simulink model "LinkageC"  (R2025b)
settings: Solver=VariableStepAuto  StartTime=0  StopTime=numPeriods*T  RelTol=1e-3  AbsTol=1e-3
values from neighbouring files (symbols this model uses):
  A_G = 56.801    [LinkageGeometrySetUp.m]    (also in LinkageGeometrySetUp_imp.m = 55; LinkageGeometry_Fabio_ver.m = 20)
  alpha_0 = deg2rad(0.5)    [Iteration.m]    (also in Iteration_geometry.m; StartUp.m)
  alpha_stall_static = deg2rad(13)    [Iteration.m]    (also in Iteration_geometry.m; StartUp.m)
  AR = b^2/A    [LinkageGeometry_Modify.m]    (also in StartUp.m)
  Cd_cf = 1.5    [Iteration.m]    (also in Iteration_geometry.m; StartUp.m)
  CordOut = linspace(CordOut_root, CordOut_tip, WingSecNum_Out)    [LinkageGeometry_Modify.m]    (also in StartUp.m)
  D = 0;" newline      "    return;" newline      "end" newline      "q = 0.5*rho*Vmag^2;" newline      "D = q*S*CD;" newline      "L = q*S*CL;" newline      "    [build_wing_template.m]
  del_t = t_tot/(numSample)    [InputSetUp.m]
  eta_s = 0.90    (= 0.9)    [Iteration.m]    (also in Iteration_geometry.m; StartUp.m)
  InboardCord = 0.35*L_D/0.037    [LinkageGeometry_Modify.m]    (also in StartUp.m = 0.4)
  k_inboard = k * InboardCord/meanCord    [LinkageGeometry_Modify.m]    (also in StartUp.m = 12.5663706144)
  k_outboard = k * CordOut/meanCord    [LinkageGeometry_Modify.m]    (also in StartUp.m)
  Ka = 10    [StartUp3_control.m]
  Km = 73    [StartUp3_control.m]
  L_C = (3.589/1.5)*L_D    [LinkageGeometrySetUp.m]    (also in LinkageGeometrySetUp_imp.m = (9.37/3.7)*L_D; LinkageGeometry_Fabio_ver.m = 0.07885)
  L_C1 = (2.445/1.5)*L_D    [LinkageGeometrySetUp.m]    (also in LinkageGeometrySetUp_imp.m = (5.91/3.7)*L_D; LinkageGeometry_Fabio_ver.m = 0.04893)
  L_D = L_D_val(iter)    [Iteration_geometry.m]    (also in LinkageGeometry_Fabio_ver.m = 0.03019; StartUp.m = 0.037)
  L_EF = (1.494/1.5)*L_D    [LinkageGeometrySetUp.m]    (also in LinkageGeometrySetUp_imp.m = (4.468/3.7)*L_D; LinkageGeometry_Fabio_ver.m = 0.036)
  L_EG = (1.265/1.5)*L_D    [LinkageGeometrySetUp.m]    (also in LinkageGeometrySetUp_imp.m = L_C2; LinkageGeometry_Fabio_ver.m = 0.03)
  L_F = (16.189/1.5)*L_D    [LinkageGeometrySetUp.m]    (also in LinkageGeometrySetUp_imp.m = (39.93/3.7)*L_D; LinkageGeometry_Fabio_ver.m = 0.364)
  L_FH = (1.002/1.5)*L_D    [LinkageGeometrySetUp.m]    (also in LinkageGeometrySetUp_imp.m = (2.842/3.7)*L_D; LinkageGeometry_Fabio_ver.m = 0.02)
  L_Fl = (16.118/1.5)*L_D    [LinkageGeometrySetUp.m]    (also in LinkageGeometrySetUp_imp.m = L_F; LinkageGeometry_Fabio_ver.m = 0.364)
  L_Fp = (4.051/1.5)*L_D    [LinkageGeometrySetUp.m]    (also in LinkageGeometrySetUp_imp.m = (9.99/3.7)*L_D; LinkageGeometry_Fabio_ver.m = 0.14288)
  L_GH = (1.129/1.5)*L_D    [LinkageGeometrySetUp.m]    (also in LinkageGeometrySetUp_imp.m = (3.046/3.7)*L_D; LinkageGeometry_Fabio_ver.m = 0.016)
  L_t = 0.5/100    (= 0.005)    [LinkageGeometrySetUp.m]    (also in LinkageGeometrySetUp_imp.m; LinkageGeometry_Fabio_ver.m; LinkageGeometry_Modify.m)
  L_tip = (19.334/1.5)*L_D    [LinkageGeometrySetUp.m]    (also in LinkageGeometrySetUp_imp.m = (43/3.7)*L_D; LinkageGeometry_Fabio_ver.m = 0.55)
  M_in_i = M_in/WingSecNum_In    (= 0.0341666666667)    [StartUp.m]
  M_ser = 0.02    [StartUp.m]
  mu = 1.81e-5    (= 1.81e-05)    [Iteration.m]    (also in Iteration_geometry.m; StartUp.m)
  noise_freq_cutoff = 20*ang_freq    [InputSetUp.m]
  P_ref = 10    [StartUp3_control.m]
  phase_data_lookup = phase_data_lookup(1:(end-1))    [StartUp.m]
  pitch_data_lookup = pitch_ts.Data(1:numSampPerT)    [InputSetUp.m]
  pitch_gain = linspace(0.1, 1, WingSecNum_Out)    [InputSetUp.m]
  pitch_lookup_input = 1    [Iteration.m]    (also in Iteration_geometry.m; StartUp.m)
  pitch_mean = deg2rad(20)    [Iteration.m]    (also in Iteration_geometry.m; Iteration_speed.m; StartUp.m = deg2rad(1); StartUp3_control.m = deg2rad(1))
  rho = 1.225    [StartUp.m]
  SectionWidth_In = L_Inboard/WingSecNum_In    [LinkageGeometry_Modify.m]    (also in StartUp.m = (L_Inboard/WingSecNum_In)*0.6)
  SectionWidth_Out = L_outboard/WingSecNum_Out    [LinkageGeometry_Modify.m]    (also in StartUp.m)
  SpeedControlYes = 1    [StartUp3_control.m]
  TorqueLimit = 7.2    [StartUp3_control.m]
  U = 0.1    [Iteration.m]    (also in Iteration_geometry.m; StartUp.m)
  xi = 0.0    (= 0)    [Iteration.m]    (also in Iteration_geometry.m; StartUp.m)
undefined symbols (not defined in the file or in its folder): angle_data_lookup, DiscIntNeverNeededParam, magnitude, Pivot, X, Y, Z
libraries: sm_lib x1370, nesl_utility x916, simulink x478, cstblocks x78, simulink_extras x10, slpidlib x2
(part 14 of 57)

== system LinkageC/Subsystem/Wing Tip/Angle ==
  PS-Simulink Converter{1..4} (4 alike) : nesl_utility/PS-Simulink Converter  PhysicalDomain=network_engine_domain  SubClassName=ps_output  LeftPortType=input  RightPortType=output  PseudoPeriodic=off  Frequencies=[]  VectorFormat=inherit  Unit=inherit  AffineConversion=off
  Radians to Degrees : simulink_extras/Transformations/Radians to Degrees
  Subtract : Sum  Inputs=+-
  Subtract1 : Sum  Inputs=+-
  To Workspace : ToWorkspace  VariableName=simout6  SampleTime=-1
  Transform Sensor : sm_lib/Frames and Transforms/Transform Sensor  MeasurementFrame=World  RotationSequence=XYX  SenseAngle=off  SenseAxis=off  SenseQ=off  SenseR=off  SenseRotationSequence=off  SenseOmegaX=off  SenseOmegaY=off  SenseOmegaZ=off  SenseOmega=off  SenseQDot=off  SenseRDot=off  SenseRotationSequenceDot=off  SenseAlphaX=off  SenseAlphaY=off  SenseAlphaZ=off  SenseAlpha=off  SenseQDDot=off  SenseRDDot=off  SenseX=on  SenseY=on  SenseZ=off  SenseXYZ=off  SenseRad=off  SenseAzim=off  SenseDist=off  SenseInc=off  SenseXDot=off  SenseYDot=off  SenseZDot=off  SenseXYZDot=off  SenseRadDot=off  SenseAzimDot=off  SenseDistDot=off  SenseIncDot=off  SenseXDDot=off  SenseYDDot=off  SenseZDDot=off  SenseXYZDDot=off  SenseRadDDot=off  SenseAzimDDot=off  SenseDistDDot=off  SenseIncDDot=off
  Transform Sensor1 : sm_lib/Frames and Transforms/Transform Sensor  MeasurementFrame=World  RotationSequence=XYX  SenseAngle=off  SenseAxis=off  SenseQ=off  SenseR=off  SenseRotationSequence=off  SenseOmegaX=off  SenseOmegaY=off  SenseOmegaZ=off  SenseOmega=off  SenseQDot=off  SenseRDot=off  SenseRotationSequenceDot=off  SenseAlphaX=off  SenseAlphaY=off  SenseAlphaZ=off  SenseAlpha=off  SenseQDDot=off  SenseRDDot=off  SenseX=on  SenseY=on  SenseZ=off  SenseXYZ=off  SenseRad=off  SenseAzim=off  SenseDist=off  SenseInc=off  SenseXDot=off  SenseYDot=off  SenseZDot=off  SenseXYZDot=off  SenseRadDot=off  SenseAzimDot=off  SenseDistDot=off  SenseIncDot=off  SenseXDDot=off  SenseYDDot=off  SenseZDDot=off  SenseXYZDDot=off  SenseRadDDot=off  SenseAzimDDot=off  SenseDistDDot=off  SenseIncDDot=off
  Trigonometric Function : Trigonometry  Operator=atan2
  World Frame : sm_lib/Frames and Transforms/World Frame
  Pivot : PMIOPort  Side=Right
  Other Frame : PMIOPort  Port=2  Side=Right
  wires:
  Subtract/1 -> Trigonometric Function/2
  PS-Simulink Converter2/1 -> Subtract1/1
  Radians to Degrees/1 -> To Workspace/1  "OB_deg"
  Subtract1/1 -> Trigonometric Function/1
  PS-Simulink Converter4/1 -> Subtract1/2
  PS-Simulink Converter3/1 -> Subtract/2
  PS-Simulink Converter1/1 -> Subtract/1
  Trigonometric Function/1 -> Radians to Degrees/1
  connections:
  PS-Simulink Converter3/LConn1 -- Transform Sensor1/RConn2
  World Frame/RConn1 -- Transform Sensor/LConn1 -- Transform Sensor1/LConn1
  Transform Sensor/RConn3 -- PS-Simulink Converter2/LConn1
  PS-Simulink Converter1/LConn1 -- Transform Sensor/RConn2
  Transform Sensor1/RConn3 -- PS-Simulink Converter4/LConn1
  Transform Sensor/RConn1 -- Other Frame/RConn1
  Transform Sensor1/RConn1 -- Pivot/RConn1

== system LinkageC/Subsystem/Wing Tip/LinkEF_discrete ==
  Subsystem : Subsystem
  Subsystem1 : Subsystem
  Subsystem2 : Subsystem
  Subsystem3 : Subsystem
  Subsystem4 : Subsystem
  Conn1 : PMIOPort  Side=Left
  Conn2 : PMIOPort  Port=2  Side=Right
  connections:
  Subsystem4/RConn1 -- Conn2/RConn1
  Subsystem/LConn1 -- Conn1/RConn1
  Subsystem2/LConn1 -- Subsystem1/RConn1
  Subsystem/RConn1 -- Subsystem1/LConn1
  Subsystem2/RConn1 -- Subsystem3/LConn1
  Subsystem4/LConn1 -- Subsystem3/RConn1

== system LinkageC/Subsystem/Wing Tip/LinkGH_discrete ==
  LinkGH_0 : Subsystem
  LinkGH_1 : Subsystem
  LinkGH_2 : Subsystem
  LinkGH_3 : Subsystem
  LinkGH_4 : Subsystem
  Pin G Pos : PMIOPort  Side=Left
  Conn2 : PMIOPort  Port=2  Side=Right
  connections:
  LinkGH_3/LConn1 -- LinkGH_2/RConn1
  LinkGH_1/RConn1 -- LinkGH_2/LConn1
  LinkGH_0/LConn1 -- Pin G Pos/RConn1
  LinkGH_3/RConn1 -- LinkGH_4/LConn1
  LinkGH_4/RConn1 -- Conn2/RConn1
  LinkGH_0/RConn1 -- LinkGH_1/LConn1

== system LinkageC/Subsystem/Wing Tip/WingSeg_Out_1 ==
  1993dL&dT : Subsystem
      settings: PortSchema="{\"entries\":[{\"content\":{\"sides\":[{\"content\":{\"connectorIds\":[\"In1\",\"In2\"]},\"type\":\"ConnectorPlacement.EquallySpacedRectSide\",\"uuid\":\"e65777f2-64e1-48f2-8a97-1c4430d49e8c\"},{\"content\":{\"connectorIds\":[\"Out1\",\"Out2\"],\"side\":\"RIGHT\"},\"type\":\"ConnectorPlacement.EquallySpacedRectSide\",\"uuid\":\"b36152b1-49d2-4fe8-8958-784e9c481724\"},{\"content\":{\"connectorIds\":[\"LConn1\"],\"side\":\"TOP\"},\"type\":\"ConnectorPlacement.EquallySpacedRectSide\",\"uuid\":\"e55ca923-aa34-4679-961a-c06571c550d8\"}]},\"type\":\"ConnectorPlacement.EquallySpacedConnector\",\"uuid\":\"74bedadb-397c-4a7f-b538-7cebaf15bb03\"}],\"packageUris\":[\"http://schema.mathworks.com/mf0/Connector/R2020b\"],\"version\":\"1.0\"}"
  Discrete Derivative : simulink/Discrete/Discrete Derivative  gainval=1.0  ICPrevScaledInput=0.0  OutMin=[]  OutMax=[]  OutDataType=fixdt(1, 16)  OutScaling=2^-10  DoSatur=off
  Discrete Derivative1 : simulink/Discrete/Discrete Derivative  gainval=1.0  ICPrevScaledInput=0.0  OutMin=[]  OutMax=[]  OutDataType=fixdt(1, 16)  OutScaling=2^-10  DoSatur=off
  DocBlock : simulink/Model-Wide Utilities/DocBlock  DocumentType=Text
      content=|
      | For each wing section, things that need to be specified includes:
      | - Wing solid dimension (use wing modify script)
      | - Wing joint gain (pitchGain, pitchGain1, pitchGain2)
      | - PivotXfm & COMXfm
      | - i value
      | - inboard_yes?
  In_yes : Constant  Value=0
  Product : Product
  Switch : Switch  Criteria=u2 > Threshold  SaturateOnIntegerOverflow=off  InputSameDT=off
  WingSolid : sm_lib/Body Elements/Brick Solid  BrickDimensions=[0.35, L_t, SectionWidth_Out]  BrickDimensionsUnits=m  ExportEntireGeometry=off  InertiaType=CalculateFromGeometry  BasedOnType=Mass  Density=1000  DensityUnits=kg/m^3  Mass=0.031429  MassUnits=kg  CenterOfMass=[0 0 0]  CenterOfMassUnits=m  MomentsOfInertia=[1 1 1]  MomentsOfInertiaUnits=kg*m^2  ProductsOfInertia=[0 0 0]  ProductsOfInertiaUnits=kg*m^2  GraphicType=FromGeometry  MarkerShape=Sphere  MarkerSize=10  GraphicVisPropType=SimpleVisualProperties  GraphicDiffuseColor=[0.37 0.4 0.8]  GraphicOpacity=1  GraphicSpecularColor=[0.5 0.5 0.5 1.0]  GraphicAmbientColor=[0.15 0.15 0.15 1.0]  GraphicEmissiveColor=[0.0 0.0 0.0 1.0]  GraphicShininess=75  DoExposeReferenceFrame=on  SerializedFrames=<Frames/>
  Wing_Joint : sm_lib/Joints/Revolute Joint  JointMode=Normal  CompositeWrenchDir=FollowerOnBase  CompositeWrenchFrame=BaseFrame  SenseConstraintForce=off  SenseConstraintTorque=off  SenseTotalForce=off  SenseTotalTorque=off  PositionTargetSpecify=off  PositionTargetPriority=High  PositionTargetValue=0  PositionTargetValueUnits=deg  VelocityTargetSpecify=off  VelocityTargetPriority=High  VelocityTargetValue=0  VelocityTargetValueUnits=deg/s  EquilibriumPosition=0  EquilibriumPositionUnits=deg  SpringStiffness=0  SpringStiffnessUnits=N*m/deg  DampingCoefficient=dampingOfJoints  DampingCoefficientUnits=N*m/(deg/s)  LowerLimitSpecify=off  LowerLimitBound=-90  LowerLimitBoundUnits=deg  LowerLimitStiffness=1e4  LowerLimitStiffnessUnits=N*m/deg  LowerLimitDamping=10  LowerLimitDampingUnits=N*m/(deg/s)  LowerLimitTransitionRegionWidth=0.1  LowerLimitTransitionRegionWidthUnits=deg  UpperLimitSpecify=off  UpperLimitBound=90  UpperLimitBoundUnits=deg  UpperLimitStiffness=1e4  UpperLimitStiffnessUnits=N*m/deg  UpperLimitDamping=10  UpperLimitDampingUnits=N*m/(deg/s)  UpperLimitTransitionRegionWidth=0.1  UpperLimitTransitionRegionWidthUnits=deg  TorqueActuationMode=ComputedTorque  MotionActuationMode=InputMotion  SensePosition=off  SenseVelocity=off  SenseAcceleration=off  SenseTorqueForce=off  SenseLowerLimitTorqueForce=off  SenseUpperLimitTorqueForce=off
  Xfm : sm_lib/Frames and Transforms/Rigid Transform  RotationMethod=None  FollAlignAxisA=+X  BaseAlignAxisA=+Y  FollAlignAxisB=+Y  BaseAlignAxisB=+Z  RotationStandardAxis=+Z  RotationAngle=0  RotationAngleUnits=deg  RotationArbitraryAxis=[0 0 1]  RotationSequenceAxes=FollowerAxes  RotationSequence=XYX  RotationSequenceAngles=[0 0 0]  RotationSequenceAnglesUnits=deg  RotationMatrix=[1 0 0;0 1 0;0 0 1]  Quaternion=[1 0 0 0]  TranslationMethod=Cartesian  TranslationCartesianOffset=[0.0875 0 0.03]  TranslationCartesianOffsetUnits=m  TranslationStandardAxis=+Z  TranslationStandardOffset=0  TranslationStandardOffsetUnits=m  TranslationROffset=0  TranslationROffsetUnits=m  TranslationThetaOffset=0  TranslationThetaOffsetUnits=deg  TranslationZOffset=0  TranslationZOffsetUnits=m
  i : Constant
  pitchGain : Gain  Gain=0.1
  pitchGain1 : Gain  Gain=0.1
  pitchGain2 : Gain  Gain=0.1
  pitchPS : nesl_utility/Simulink-PS Converter  PhysicalDomain=network_engine_domain  SubClassName=ps_input  LeftPortType=input  RightPortType=output  PseudoPeriodic=off  Frequencies=[]  NoiseDistribution=none  NoiseParameters=[]  Unit=rad  AffineConversion=off  FilteringAndDerivatives=provide  SimscapeFilterOrder=1  InputFilterTimeConstant=0.001  UdotUserProvided=2
  pitch_lookup?(1=yes) : Constant  Value=pitch_lookup_input
  pitch_tip_in : FromWorkspace  VariableName=pitch_tip_in  SampleTime=del_t
  simulation sign convention differ : Constant  Value=-1
  WingRef_Frame : PMIOPort  Side=Left
  dL : Outport
  dT : Outport  Port=2
  wires:
  pitch_tip_in/1 -> Switch/3  "pitch"
  [pitch_m] -> Switch/1
  Switch/1 -> Product/1
  pitch_lookup?(1=yes)/1 -> Switch/2
  Product/1 -> pitchGain/1, Discrete Derivative/1
  simulation sign convention differ/1 -> Product/2
  In_yes/1 -> 1993dL&dT/2(inboard_yes?)
  i/1 -> 1993dL&dT/1(i)
  1993dL&dT/2(dT) -> dT/1
  Discrete Derivative/1 -> pitchGain1/1, Discrete Derivative1/1
  pitchGain/1 -> pitchPS/1
  1993dL&dT/1(dL) -> dL/1
  pitchGain2/1 -> pitchPS/3
  Discrete Derivative1/1 -> pitchGain2/1  "acc"
  pitchGain1/1 -> pitchPS/2
  connections:
  Xfm/LConn1 -- Wing_Joint/RConn1
  1993dL&dT/LConn1 -- Xfm/RConn1 -- WingSolid/RConn1
  pitchPS/RConn1 -- Wing_Joint/LConn2
  Wing_Joint/LConn1 -- WingRef_Frame/RConn1

== system LinkageC/Subsystem/Wing Tip/WingSeg_Out_10 ==
  1993dL&dT : Subsystem
      settings: PortSchema="{\"entries\":[{\"content\":{\"sides\":[{\"content\":{\"connectorIds\":[\"In1\",\"In2\"]},\"type\":\"ConnectorPlacement.EquallySpacedRectSide\",\"uuid\":\"e65777f2-64e1-48f2-8a97-1c4430d49e8c\"},{\"content\":{\"connectorIds\":[\"Out1\",\"Out2\"],\"side\":\"RIGHT\"},\"type\":\"ConnectorPlacement.EquallySpacedRectSide\",\"uuid\":\"b36152b1-49d2-4fe8-8958-784e9c481724\"},{\"content\":{\"connectorIds\":[\"LConn1\"],\"side\":\"TOP\"},\"type\":\"ConnectorPlacement.EquallySpacedRectSide\",\"uuid\":\"e55ca923-aa34-4679-961a-c06571c550d8\"}]},\"type\":\"ConnectorPlacement.EquallySpacedConnector\",\"uuid\":\"74bedadb-397c-4a7f-b538-7cebaf15bb03\"}],\"packageUris\":[\"http://schema.mathworks.com/mf0/Connector/R2020b\"],\"version\":\"1.0\"}"
  Discrete Derivative : simulink/Discrete/Discrete Derivative  gainval=1.0  ICPrevScaledInput=0.0  OutMin=[]  OutMax=[]  OutDataType=fixdt(1, 16)  OutScaling=2^-10  DoSatur=off
  Discrete Derivative1 : simulink/Discrete/Discrete Derivative  gainval=1.0  ICPrevScaledInput=0.0  OutMin=[]  OutMax=[]  OutDataType=fixdt(1, 16)  OutScaling=2^-10  DoSatur=off
  DocBlock : simulink/Model-Wide Utilities/DocBlock  DocumentType=Text
      content=|
      | For each wing section, things that need to be specified includes:
      | - Wing solid dimension (use wing modify script)
      | - Wing joint gain (pitchGain, pitchGain1, pitchGain2)
      | - PivotXfm & COMXfm
      | - i value
      | - inboard_yes?
  In_yes : Constant  Value=0
  Product : Product
  Switch : Switch  Criteria=u2 > Threshold  SaturateOnIntegerOverflow=off  InputSameDT=off
  WingSolid : sm_lib/Body Elements/Brick Solid  BrickDimensions=[0.14, L_t, SectionWidth_Out]  BrickDimensionsUnits=m  ExportEntireGeometry=off  InertiaType=CalculateFromGeometry  BasedOnType=Mass  Density=1000  DensityUnits=kg/m^3  Mass=0.012571  MassUnits=kg  CenterOfMass=[0 0 0]  CenterOfMassUnits=m  MomentsOfInertia=[1 1 1]  MomentsOfInertiaUnits=kg*m^2  ProductsOfInertia=[0 0 0]  ProductsOfInertiaUnits=kg*m^2  GraphicType=FromGeometry  MarkerShape=Sphere  MarkerSize=10  GraphicVisPropType=SimpleVisualProperties  GraphicDiffuseColor=[1 0.4 0.8]  GraphicOpacity=1  GraphicSpecularColor=[0.5 0.5 0.5 1.0]  GraphicAmbientColor=[0.15 0.15 0.15 1.0]  GraphicEmissiveColor=[0.0 0.0 0.0 1.0]  GraphicShininess=75  DoExposeReferenceFrame=on  SerializedFrames=<Frames/>
  Wing_Joint : sm_lib/Joints/Revolute Joint  JointMode=Normal  CompositeWrenchDir=FollowerOnBase  CompositeWrenchFrame=BaseFrame  SenseConstraintForce=off  SenseConstraintTorque=off  SenseTotalForce=off  SenseTotalTorque=off  PositionTargetSpecify=off  PositionTargetPriority=High  PositionTargetValue=0  PositionTargetValueUnits=deg  VelocityTargetSpecify=off  VelocityTargetPriority=High  VelocityTargetValue=0  VelocityTargetValueUnits=deg/s  EquilibriumPosition=0  EquilibriumPositionUnits=deg  SpringStiffness=0  SpringStiffnessUnits=N*m/deg  DampingCoefficient=dampingOfJoints  DampingCoefficientUnits=N*m/(deg/s)  LowerLimitSpecify=off  LowerLimitBound=-90  LowerLimitBoundUnits=deg  LowerLimitStiffness=1e4  LowerLimitStiffnessUnits=N*m/deg  LowerLimitDamping=10  LowerLimitDampingUnits=N*m/(deg/s)  LowerLimitTransitionRegionWidth=0.1  LowerLimitTransitionRegionWidthUnits=deg  UpperLimitSpecify=off  UpperLimitBound=90  UpperLimitBoundUnits=deg  UpperLimitStiffness=1e4  UpperLimitStiffnessUnits=N*m/deg  UpperLimitDamping=10  UpperLimitDampingUnits=N*m/(deg/s)  UpperLimitTransitionRegionWidth=0.1  UpperLimitTransitionRegionWidthUnits=deg  TorqueActuationMode=ComputedTorque  MotionActuationMode=InputMotion  SensePosition=off  SenseVelocity=off  SenseAcceleration=off  SenseTorqueForce=off  SenseLowerLimitTorqueForce=off  SenseUpperLimitTorqueForce=off
  Xfm : sm_lib/Frames and Transforms/Rigid Transform  RotationMethod=None  FollAlignAxisA=+X  BaseAlignAxisA=+Y  FollAlignAxisB=+Y  BaseAlignAxisB=+Z  RotationStandardAxis=+Z  RotationAngle=0  RotationAngleUnits=deg  RotationArbitraryAxis=[0 0 1]  RotationSequenceAxes=FollowerAxes  RotationSequence=XYX  RotationSequenceAngles=[0 0 0]  RotationSequenceAnglesUnits=deg  RotationMatrix=[1 0 0;0 1 0;0 0 1]  Quaternion=[1 0 0 0]  TranslationMethod=Cartesian  TranslationCartesianOffset=[0.035 0 0.57]  TranslationCartesianOffsetUnits=m  TranslationStandardAxis=+Z  TranslationStandardOffset=0  TranslationStandardOffsetUnits=m  TranslationROffset=0  TranslationROffsetUnits=m  TranslationThetaOffset=0  TranslationThetaOffsetUnits=deg  TranslationZOffset=0  TranslationZOffsetUnits=m
  i : Constant  Value=10
  pitchGain : Gain
  pitchGain1 : Gain
  pitchGain2 : Gain
  pitchPS : nesl_utility/Simulink-PS Converter  PhysicalDomain=network_engine_domain  SubClassName=ps_input  LeftPortType=input  RightPortType=output  PseudoPeriodic=off  Frequencies=[]  NoiseDistribution=none  NoiseParameters=[]  Unit=rad  AffineConversion=off  FilteringAndDerivatives=provide  SimscapeFilterOrder=1  InputFilterTimeConstant=0.001  UdotUserProvided=2
  pitch_lookup?(1=yes) : Constant  Value=pitch_lookup_input
  pitch_tip_in : FromWorkspace  VariableName=pitch_tip_in  SampleTime=del_t
  simulation sign convention differ : Constant  Value=-1
  WingRef_Frame : PMIOPort  Side=Left
  dL : Outport
  dT : Outport  Port=2
  wires:
  pitch_tip_in/1 -> Switch/3  "pitch"
  [pitch_m] -> Switch/1
  Switch/1 -> Product/1
  pitch_lookup?(1=yes)/1 -> Switch/2
  Product/1 -> pitchGain/1, Discrete Derivative/1
  simulation sign convention differ/1 -> Product/2
  In_yes/1 -> 1993dL&dT/2(inboard_yes?)
  i/1 -> 1993dL&dT/1(i)
  1993dL&dT/2(dT) -> dT/1
  Discrete Derivative/1 -> pitchGain1/1, Discrete Derivative1/1
  pitchGain/1 -> pitchPS/1
  1993dL&dT/1(dL) -> dL/1
  pitchGain2/1 -> pitchPS/3
  Discrete Derivative1/1 -> pitchGain2/1  "acc"
  pitchGain1/1 -> pitchPS/2
  connections:
  Xfm/LConn1 -- Wing_Joint/RConn1
  1993dL&dT/LConn1 -- Xfm/RConn1 -- WingSolid/RConn1
  pitchPS/RConn1 -- Wing_Joint/LConn2
  Wing_Joint/LConn1 -- WingRef_Frame/RConn1

== system LinkageC/Subsystem/Wing Tip/WingSeg_Out_2 ==
  1993dL&dT : Subsystem
      settings: PortSchema="{\"entries\":[{\"content\":{\"sides\":[{\"content\":{\"connectorIds\":[\"In1\",\"In2\"]},\"type\":\"ConnectorPlacement.EquallySpacedRectSide\",\"uuid\":\"e65777f2-64e1-48f2-8a97-1c4430d49e8c\"},{\"content\":{\"connectorIds\":[\"Out1\",\"Out2\"],\"side\":\"RIGHT\"},\"type\":\"ConnectorPlacement.EquallySpacedRectSide\",\"uuid\":\"b36152b1-49d2-4fe8-8958-784e9c481724\"},{\"content\":{\"connectorIds\":[\"LConn1\"],\"side\":\"TOP\"},\"type\":\"ConnectorPlacement.EquallySpacedRectSide\",\"uuid\":\"e55ca923-aa34-4679-961a-c06571c550d8\"}]},\"type\":\"ConnectorPlacement.EquallySpacedConnector\",\"uuid\":\"74bedadb-397c-4a7f-b538-7cebaf15bb03\"}],\"packageUris\":[\"http://schema.mathworks.com/mf0/Connector/R2020b\"],\"version\":\"1.0\"}"
  Discrete Derivative : simulink/Discrete/Discrete Derivative  gainval=1.0  ICPrevScaledInput=0.0  OutMin=[]  OutMax=[]  OutDataType=fixdt(1, 16)  OutScaling=2^-10  DoSatur=off
  Discrete Derivative1 : simulink/Discrete/Discrete Derivative  gainval=1.0  ICPrevScaledInput=0.0  OutMin=[]  OutMax=[]  OutDataType=fixdt(1, 16)  OutScaling=2^-10  DoSatur=off
  DocBlock : simulink/Model-Wide Utilities/DocBlock  DocumentType=Text
      content=|
      | For each wing section, things that need to be specified includes:
      | - Wing solid dimension (use wing modify script)
      | - Wing joint gain (pitchGain, pitchGain1, pitchGain2)
      | - PivotXfm & COMXfm
      | - i value
      | - inboard_yes?
  In_yes : Constant  Value=0
  Product : Product
  Switch : Switch  Criteria=u2 > Threshold  SaturateOnIntegerOverflow=off  InputSameDT=off
  WingSolid : sm_lib/Body Elements/Brick Solid  BrickDimensions=[0.32667, L_t, SectionWidth_Out]  BrickDimensionsUnits=m  ExportEntireGeometry=off  InertiaType=CalculateFromGeometry  BasedOnType=Mass  Density=1000  DensityUnits=kg/m^3  Mass=0.029333  MassUnits=kg  CenterOfMass=[0 0 0]  CenterOfMassUnits=m  MomentsOfInertia=[1 1 1]  MomentsOfInertiaUnits=kg*m^2  ProductsOfInertia=[0 0 0]  ProductsOfInertiaUnits=kg*m^2  GraphicType=FromGeometry  MarkerShape=Sphere  MarkerSize=10  GraphicVisPropType=SimpleVisualProperties  GraphicDiffuseColor=[0.44 0.4 0.8]  GraphicOpacity=1  GraphicSpecularColor=[0.5 0.5 0.5 1.0]  GraphicAmbientColor=[0.15 0.15 0.15 1.0]  GraphicEmissiveColor=[0.0 0.0 0.0 1.0]  GraphicShininess=75  DoExposeReferenceFrame=on  SerializedFrames=<Frames/>
  Wing_Joint : sm_lib/Joints/Revolute Joint  JointMode=Normal  CompositeWrenchDir=FollowerOnBase  CompositeWrenchFrame=BaseFrame  SenseConstraintForce=off  SenseConstraintTorque=off  SenseTotalForce=off  SenseTotalTorque=off  PositionTargetSpecify=off  PositionTargetPriority=High  PositionTargetValue=0  PositionTargetValueUnits=deg  VelocityTargetSpecify=off  VelocityTargetPriority=High  VelocityTargetValue=0  VelocityTargetValueUnits=deg/s  EquilibriumPosition=0  EquilibriumPositionUnits=deg  SpringStiffness=0  SpringStiffnessUnits=N*m/deg  DampingCoefficient=dampingOfJoints  DampingCoefficientUnits=N*m/(deg/s)  LowerLimitSpecify=off  LowerLimitBound=-90  LowerLimitBoundUnits=deg  LowerLimitStiffness=1e4  LowerLimitStiffnessUnits=N*m/deg  LowerLimitDamping=10  LowerLimitDampingUnits=N*m/(deg/s)  LowerLimitTransitionRegionWidth=0.1  LowerLimitTransitionRegionWidthUnits=deg  UpperLimitSpecify=off  UpperLimitBound=90  UpperLimitBoundUnits=deg  UpperLimitStiffness=1e4  UpperLimitStiffnessUnits=N*m/deg  UpperLimitDamping=10  UpperLimitDampingUnits=N*m/(deg/s)  UpperLimitTransitionRegionWidth=0.1  UpperLimitTransitionRegionWidthUnits=deg  TorqueActuationMode=ComputedTorque  MotionActuationMode=InputMotion  SensePosition=off  SenseVelocity=off  SenseAcceleration=off  SenseTorqueForce=off  SenseLowerLimitTorqueForce=off  SenseUpperLimitTorqueForce=off
  Xfm : sm_lib/Frames and Transforms/Rigid Transform  RotationMethod=None  FollAlignAxisA=+X  BaseAlignAxisA=+Y  FollAlignAxisB=+Y  BaseAlignAxisB=+Z  RotationStandardAxis=+Z  RotationAngle=0  RotationAngleUnits=deg  RotationArbitraryAxis=[0 0 1]  RotationSequenceAxes=FollowerAxes  RotationSequence=XYX  RotationSequenceAngles=[0 0 0]  RotationSequenceAnglesUnits=deg  RotationMatrix=[1 0 0;0 1 0;0 0 1]  Quaternion=[1 0 0 0]  TranslationMethod=Cartesian  TranslationCartesianOffset=[0.081667 0 0.09]  TranslationCartesianOffsetUnits=m  TranslationStandardAxis=+Z  TranslationStandardOffset=0  TranslationStandardOffsetUnits=m  TranslationROffset=0  TranslationROffsetUnits=m  TranslationThetaOffset=0  TranslationThetaOffsetUnits=deg  TranslationZOffset=0  TranslationZOffsetUnits=m
  i : Constant  Value=2
  pitchGain : Gain  Gain=0.2
  pitchGain1 : Gain  Gain=0.2
  pitchGain2 : Gain  Gain=0.2
  pitchPS : nesl_utility/Simulink-PS Converter  PhysicalDomain=network_engine_domain  SubClassName=ps_input  LeftPortType=input  RightPortType=output  PseudoPeriodic=off  Frequencies=[]  NoiseDistribution=none  NoiseParameters=[]  Unit=rad  AffineConversion=off  FilteringAndDerivatives=provide  SimscapeFilterOrder=1  InputFilterTimeConstant=0.001  UdotUserProvided=2
  pitch_lookup?(1=yes) : Constant  Value=pitch_lookup_input
  pitch_tip_in : FromWorkspace  VariableName=pitch_tip_in  SampleTime=del_t
  simulation sign convention differ : Constant  Value=-1
  WingRef_Frame : PMIOPort  Side=Left
  dL : Outport
  dT : Outport  Port=2
  wires:
  pitch_tip_in/1 -> Switch/3  "pitch"
  [pitch_m] -> Switch/1
  Switch/1 -> Product/1
  pitch_lookup?(1=yes)/1 -> Switch/2
  Product/1 -> pitchGain/1, Discrete Derivative/1
  simulation sign convention differ/1 -> Product/2
  In_yes/1 -> 1993dL&dT/2(inboard_yes?)
  i/1 -> 1993dL&dT/1(i)
  1993dL&dT/2(dT) -> dT/1
  Discrete Derivative/1 -> pitchGain1/1, Discrete Derivative1/1
  pitchGain/1 -> pitchPS/1
  1993dL&dT/1(dL) -> dL/1
  pitchGain2/1 -> pitchPS/3
  Discrete Derivative1/1 -> pitchGain2/1  "acc"
  pitchGain1/1 -> pitchPS/2
  connections:
  Xfm/LConn1 -- Wing_Joint/RConn1
  1993dL&dT/LConn1 -- Xfm/RConn1 -- WingSolid/RConn1
  pitchPS/RConn1 -- Wing_Joint/LConn2
  Wing_Joint/LConn1 -- WingRef_Frame/RConn1

== system LinkageC/Subsystem/Wing Tip/WingSeg_Out_3 ==
  1993dL&dT : Subsystem
      settings: PortSchema="{\"entries\":[{\"content\":{\"sides\":[{\"content\":{\"connectorIds\":[\"In1\",\"In2\"]},\"type\":\"ConnectorPlacement.EquallySpacedRectSide\",\"uuid\":\"e65777f2-64e1-48f2-8a97-1c4430d49e8c\"},{\"content\":{\"connectorIds\":[\"Out1\",\"Out2\"],\"side\":\"RIGHT\"},\"type\":\"ConnectorPlacement.EquallySpacedRectSide\",\"uuid\":\"b36152b1-49d2-4fe8-8958-784e9c481724\"},{\"content\":{\"connectorIds\":[\"LConn1\"],\"side\":\"TOP\"},\"type\":\"ConnectorPlacement.EquallySpacedRectSide\",\"uuid\":\"e55ca923-aa34-4679-961a-c06571c550d8\"}]},\"type\":\"ConnectorPlacement.EquallySpacedConnector\",\"uuid\":\"74bedadb-397c-4a7f-b538-7cebaf15bb03\"}],\"packageUris\":[\"http://schema.mathworks.com/mf0/Connector/R2020b\"],\"version\":\"1.0\"}"
  Discrete Derivative : simulink/Discrete/Discrete Derivative  gainval=1.0  ICPrevScaledInput=0.0  OutMin=[]  OutMax=[]  OutDataType=fixdt(1, 16)  OutScaling=2^-10  DoSatur=off
  Discrete Derivative1 : simulink/Discrete/Discrete Derivative  gainval=1.0  ICPrevScaledInput=0.0  OutMin=[]  OutMax=[]  OutDataType=fixdt(1, 16)  OutScaling=2^-10  DoSatur=off
  DocBlock : simulink/Model-Wide Utilities/DocBlock  DocumentType=Text
      content=|
      | For each wing section, things that need to be specified includes:
      | - Wing solid dimension (use wing modify script)
      | - Wing joint gain (pitchGain, pitchGain1, pitchGain2)
      | - PivotXfm & COMXfm
      | - i value
      | - inboard_yes?
  In_yes : Constant  Value=0
  Product : Product
  Switch : Switch  Criteria=u2 > Threshold  SaturateOnIntegerOverflow=off  InputSameDT=off
  WingSolid : sm_lib/Body Elements/Brick Solid  BrickDimensions=[0.30333, L_t, SectionWidth_Out]  BrickDimensionsUnits=m  ExportEntireGeometry=off  InertiaType=CalculateFromGeometry  BasedOnType=Mass  Density=1000  DensityUnits=kg/m^3  Mass=0.027238  MassUnits=kg  CenterOfMass=[0 0 0]  CenterOfMassUnits=m  MomentsOfInertia=[1 1 1]  MomentsOfInertiaUnits=kg*m^2  ProductsOfInertia=[0 0 0]  ProductsOfInertiaUnits=kg*m^2  GraphicType=FromGeometry  MarkerShape=Sphere  MarkerSize=10  GraphicVisPropType=SimpleVisualProperties  GraphicDiffuseColor=[0.51 0.4 0.8]  GraphicOpacity=1  GraphicSpecularColor=[0.5 0.5 0.5 1.0]  GraphicAmbientColor=[0.15 0.15 0.15 1.0]  GraphicEmissiveColor=[0.0 0.0 0.0 1.0]  GraphicShininess=75  DoExposeReferenceFrame=on  SerializedFrames=<Frames/>
  Wing_Joint : sm_lib/Joints/Revolute Joint  JointMode=Normal  CompositeWrenchDir=FollowerOnBase  CompositeWrenchFrame=BaseFrame  SenseConstraintForce=off  SenseConstraintTorque=off  SenseTotalForce=off  SenseTotalTorque=off  PositionTargetSpecify=off  PositionTargetPriority=High  PositionTargetValue=0  PositionTargetValueUnits=deg  VelocityTargetSpecify=off  VelocityTargetPriority=High  VelocityTargetValue=0  VelocityTargetValueUnits=deg/s  EquilibriumPosition=0  EquilibriumPositionUnits=deg  SpringStiffness=0  SpringStiffnessUnits=N*m/deg  DampingCoefficient=dampingOfJoints  DampingCoefficientUnits=N*m/(deg/s)  LowerLimitSpecify=off  LowerLimitBound=-90  LowerLimitBoundUnits=deg  LowerLimitStiffness=1e4  LowerLimitStiffnessUnits=N*m/deg  LowerLimitDamping=10  LowerLimitDampingUnits=N*m/(deg/s)  LowerLimitTransitionRegionWidth=0.1  LowerLimitTransitionRegionWidthUnits=deg  UpperLimitSpecify=off  UpperLimitBound=90  UpperLimitBoundUnits=deg  UpperLimitStiffness=1e4  UpperLimitStiffnessUnits=N*m/deg  UpperLimitDamping=10  UpperLimitDampingUnits=N*m/(deg/s)  UpperLimitTransitionRegionWidth=0.1  UpperLimitTransitionRegionWidthUnits=deg  TorqueActuationMode=ComputedTorque  MotionActuationMode=InputMotion  SensePosition=off  SenseVelocity=off  SenseAcceleration=off  SenseTorqueForce=off  SenseLowerLimitTorqueForce=off  SenseUpperLimitTorqueForce=off
  Xfm : sm_lib/Frames and Transforms/Rigid Transform  RotationMethod=None  FollAlignAxisA=+X  BaseAlignAxisA=+Y  FollAlignAxisB=+Y  BaseAlignAxisB=+Z  RotationStandardAxis=+Z  RotationAngle=0  RotationAngleUnits=deg  RotationArbitraryAxis=[0 0 1]  RotationSequenceAxes=FollowerAxes  RotationSequence=XYX  RotationSequenceAngles=[0 0 0]  RotationSequenceAnglesUnits=deg  RotationMatrix=[1 0 0;0 1 0;0 0 1]  Quaternion=[1 0 0 0]  TranslationMethod=Cartesian  TranslationCartesianOffset=[0.075833 0 0.15]  TranslationCartesianOffsetUnits=m  TranslationStandardAxis=+Z  TranslationStandardOffset=0  TranslationStandardOffsetUnits=m  TranslationROffset=0  TranslationROffsetUnits=m  TranslationThetaOffset=0  TranslationThetaOffsetUnits=deg  TranslationZOffset=0  TranslationZOffsetUnits=m
  i : Constant  Value=3
  pitchGain : Gain  Gain=0.3
  pitchGain1 : Gain  Gain=0.3
  pitchGain2 : Gain  Gain=0.3
  pitchPS : nesl_utility/Simulink-PS Converter  PhysicalDomain=network_engine_domain  SubClassName=ps_input  LeftPortType=input  RightPortType=output  PseudoPeriodic=off  Frequencies=[]  NoiseDistribution=none  NoiseParameters=[]  Unit=rad  AffineConversion=off  FilteringAndDerivatives=provide  SimscapeFilterOrder=1  InputFilterTimeConstant=0.001  UdotUserProvided=2
  pitch_lookup?(1=yes) : Constant  Value=pitch_lookup_input
  pitch_tip_in : FromWorkspace  VariableName=pitch_tip_in  SampleTime=del_t
  simulation sign convention differ : Constant  Value=-1
  WingRef_Frame : PMIOPort  Side=Left
  dL : Outport
  dT : Outport  Port=2
  wires:
  pitch_tip_in/1 -> Switch/3  "pitch"
  [pitch_m] -> Switch/1
  Switch/1 -> Product/1
  pitch_lookup?(1=yes)/1 -> Switch/2
  Product/1 -> pitchGain/1, Discrete Derivative/1
  simulation sign convention differ/1 -> Product/2
  In_yes/1 -> 1993dL&dT/2(inboard_yes?)
  i/1 -> 1993dL&dT/1(i)
  1993dL&dT/2(dT) -> dT/1
  Discrete Derivative/1 -> pitchGain1/1, Discrete Derivative1/1
  pitchGain/1 -> pitchPS/1
  1993dL&dT/1(dL) -> dL/1
  pitchGain2/1 -> pitchPS/3
  Discrete Derivative1/1 -> pitchGain2/1  "acc"
  pitchGain1/1 -> pitchPS/2
  connections:
  Xfm/LConn1 -- Wing_Joint/RConn1
  1993dL&dT/LConn1 -- Xfm/RConn1 -- WingSolid/RConn1
  pitchPS/RConn1 -- Wing_Joint/LConn2
  Wing_Joint/LConn1 -- WingRef_Frame/RConn1

== system LinkageC/Subsystem/Wing Tip/WingSeg_Out_4 ==
  1993dL&dT : Subsystem
      settings: PortSchema="{\"entries\":[{\"content\":{\"sides\":[{\"content\":{\"connectorIds\":[\"In1\",\"In2\"]},\"type\":\"ConnectorPlacement.EquallySpacedRectSide\",\"uuid\":\"e65777f2-64e1-48f2-8a97-1c4430d49e8c\"},{\"content\":{\"connectorIds\":[\"Out1\",\"Out2\"],\"side\":\"RIGHT\"},\"type\":\"ConnectorPlacement.EquallySpacedRectSide\",\"uuid\":\"b36152b1-49d2-4fe8-8958-784e9c481724\"},{\"content\":{\"connectorIds\":[\"LConn1\"],\"side\":\"TOP\"},\"type\":\"ConnectorPlacement.EquallySpacedRectSide\",\"uuid\":\"e55ca923-aa34-4679-961a-c06571c550d8\"}]},\"type\":\"ConnectorPlacement.EquallySpacedConnector\",\"uuid\":\"74bedadb-397c-4a7f-b538-7cebaf15bb03\"}],\"packageUris\":[\"http://schema.mathworks.com/mf0/Connector/R2020b\"],\"version\":\"1.0\"}"
  Discrete Derivative : simulink/Discrete/Discrete Derivative  gainval=1.0  ICPrevScaledInput=0.0  OutMin=[]  OutMax=[]  OutDataType=fixdt(1, 16)  OutScaling=2^-10  DoSatur=off
  Discrete Derivative1 : simulink/Discrete/Discrete Derivative  gainval=1.0  ICPrevScaledInput=0.0  OutMin=[]  OutMax=[]  OutDataType=fixdt(1, 16)  OutScaling=2^-10  DoSatur=off
  DocBlock : simulink/Model-Wide Utilities/DocBlock  DocumentType=Text
      content=|
      | For each wing section, things that need to be specified includes:
      | - Wing solid dimension (use wing modify script)
      | - Wing joint gain (pitchGain, pitchGain1, pitchGain2)
      | - PivotXfm & COMXfm
      | - i value
      | - inboard_yes?
  In_yes : Constant  Value=0
  Product : Product
  Switch : Switch  Criteria=u2 > Threshold  SaturateOnIntegerOverflow=off  InputSameDT=off
  WingSolid : sm_lib/Body Elements/Brick Solid  BrickDimensions=[0.28, L_t, SectionWidth_Out]  BrickDimensionsUnits=m  ExportEntireGeometry=off  InertiaType=CalculateFromGeometry  BasedOnType=Mass  Density=1000  DensityUnits=kg/m^3  Mass=0.025143  MassUnits=kg  CenterOfMass=[0 0 0]  CenterOfMassUnits=m  MomentsOfInertia=[1 1 1]  MomentsOfInertiaUnits=kg*m^2  ProductsOfInertia=[0 0 0]  ProductsOfInertiaUnits=kg*m^2  GraphicType=FromGeometry  MarkerShape=Sphere  MarkerSize=10  GraphicVisPropType=SimpleVisualProperties  GraphicDiffuseColor=[0.58 0.4 0.8]  GraphicOpacity=1  GraphicSpecularColor=[0.5 0.5 0.5 1.0]  GraphicAmbientColor=[0.15 0.15 0.15 1.0]  GraphicEmissiveColor=[0.0 0.0 0.0 1.0]  GraphicShininess=75  DoExposeReferenceFrame=on  SerializedFrames=<Frames/>
  Wing_Joint : sm_lib/Joints/Revolute Joint  JointMode=Normal  CompositeWrenchDir=FollowerOnBase  CompositeWrenchFrame=BaseFrame  SenseConstraintForce=off  SenseConstraintTorque=off  SenseTotalForce=off  SenseTotalTorque=off  PositionTargetSpecify=off  PositionTargetPriority=High  PositionTargetValue=0  PositionTargetValueUnits=deg  VelocityTargetSpecify=off  VelocityTargetPriority=High  VelocityTargetValue=0  VelocityTargetValueUnits=deg/s  EquilibriumPosition=0  EquilibriumPositionUnits=deg  SpringStiffness=0  SpringStiffnessUnits=N*m/deg  DampingCoefficient=dampingOfJoints  DampingCoefficientUnits=N*m/(deg/s)  LowerLimitSpecify=off  LowerLimitBound=-90  LowerLimitBoundUnits=deg  LowerLimitStiffness=1e4  LowerLimitStiffnessUnits=N*m/deg  LowerLimitDamping=10  LowerLimitDampingUnits=N*m/(deg/s)  LowerLimitTransitionRegionWidth=0.1  LowerLimitTransitionRegionWidthUnits=deg  UpperLimitSpecify=off  UpperLimitBound=90  UpperLimitBoundUnits=deg  UpperLimitStiffness=1e4  UpperLimitStiffnessUnits=N*m/deg  UpperLimitDamping=10  UpperLimitDampingUnits=N*m/(deg/s)  UpperLimitTransitionRegionWidth=0.1  UpperLimitTransitionRegionWidthUnits=deg  TorqueActuationMode=ComputedTorque  MotionActuationMode=InputMotion  SensePosition=off  SenseVelocity=off  SenseAcceleration=off  SenseTorqueForce=off  SenseLowerLimitTorqueForce=off  SenseUpperLimitTorqueForce=off
  Xfm : sm_lib/Frames and Transforms/Rigid Transform  RotationMethod=None  FollAlignAxisA=+X  BaseAlignAxisA=+Y  FollAlignAxisB=+Y  BaseAlignAxisB=+Z  RotationStandardAxis=+Z  RotationAngle=0  RotationAngleUnits=deg  RotationArbitraryAxis=[0 0 1]  RotationSequenceAxes=FollowerAxes  RotationSequence=XYX  RotationSequenceAngles=[0 0 0]  RotationSequenceAnglesUnits=deg  RotationMatrix=[1 0 0;0 1 0;0 0 1]  Quaternion=[1 0 0 0]  TranslationMethod=Cartesian  TranslationCartesianOffset=[0.07 0 0.21]  TranslationCartesianOffsetUnits=m  TranslationStandardAxis=+Z  TranslationStandardOffset=0  TranslationStandardOffsetUnits=m  TranslationROffset=0  TranslationROffsetUnits=m  TranslationThetaOffset=0  TranslationThetaOffsetUnits=deg  TranslationZOffset=0  TranslationZOffsetUnits=m
  i : Constant  Value=4
  pitchGain : Gain  Gain=0.4
  pitchGain1 : Gain  Gain=0.4
  pitchGain2 : Gain  Gain=0.4
  pitchPS : nesl_utility/Simulink-PS Converter  PhysicalDomain=network_engine_domain  SubClassName=ps_input  LeftPortType=input  RightPortType=output  PseudoPeriodic=off  Frequencies=[]  NoiseDistribution=none  NoiseParameters=[]  Unit=rad  AffineConversion=off  FilteringAndDerivatives=provide  SimscapeFilterOrder=1  InputFilterTimeConstant=0.001  UdotUserProvided=2
  pitch_lookup?(1=yes) : Constant  Value=pitch_lookup_input
  pitch_tip_in : FromWorkspace  VariableName=pitch_tip_in  SampleTime=del_t
  simulation sign convention differ : Constant  Value=-1
  WingRef_Frame : PMIOPort  Side=Left
  dL : Outport
  dT : Outport  Port=2
  wires:
  pitch_tip_in/1 -> Switch/3  "pitch"
  [pitch_m] -> Switch/1
  Switch/1 -> Product/1
  pitch_lookup?(1=yes)/1 -> Switch/2
  Product/1 -> pitchGain/1, Discrete Derivative/1
  simulation sign convention differ/1 -> Product/2
  In_yes/1 -> 1993dL&dT/2(inboard_yes?)
  i/1 -> 1993dL&dT/1(i)
  1993dL&dT/2(dT) -> dT/1
  Discrete Derivative/1 -> pitchGain1/1, Discrete Derivative1/1
  pitchGain/1 -> pitchPS/1
  1993dL&dT/1(dL) -> dL/1
  pitchGain2/1 -> pitchPS/3
  Discrete Derivative1/1 -> pitchGain2/1  "acc"
  pitchGain1/1 -> pitchPS/2
  connections:
  Xfm/LConn1 -- Wing_Joint/RConn1
  1993dL&dT/LConn1 -- Xfm/RConn1 -- WingSolid/RConn1
  pitchPS/RConn1 -- Wing_Joint/LConn2
  Wing_Joint/LConn1 -- WingRef_Frame/RConn1

== system LinkageC/Subsystem/Wing Tip/WingSeg_Out_5 ==
  1993dL&dT : Subsystem
      settings: PortSchema="{\"entries\":[{\"content\":{\"sides\":[{\"content\":{\"connectorIds\":[\"In1\",\"In2\"]},\"type\":\"ConnectorPlacement.EquallySpacedRectSide\",\"uuid\":\"e65777f2-64e1-48f2-8a97-1c4430d49e8c\"},{\"content\":{\"connectorIds\":[\"Out1\",\"Out2\"],\"side\":\"RIGHT\"},\"type\":\"ConnectorPlacement.EquallySpacedRectSide\",\"uuid\":\"b36152b1-49d2-4fe8-8958-784e9c481724\"},{\"content\":{\"connectorIds\":[\"LConn1\"],\"side\":\"TOP\"},\"type\":\"ConnectorPlacement.EquallySpacedRectSide\",\"uuid\":\"e55ca923-aa34-4679-961a-c06571c550d8\"}]},\"type\":\"ConnectorPlacement.EquallySpacedConnector\",\"uuid\":\"74bedadb-397c-4a7f-b538-7cebaf15bb03\"}],\"packageUris\":[\"http://schema.mathworks.com/mf0/Connector/R2020b\"],\"version\":\"1.0\"}"
  Discrete Derivative : simulink/Discrete/Discrete Derivative  gainval=1.0  ICPrevScaledInput=0.0  OutMin=[]  OutMax=[]  OutDataType=fixdt(1, 16)  OutScaling=2^-10  DoSatur=off
  Discrete Derivative1 : simulink/Discrete/Discrete Derivative  gainval=1.0  ICPrevScaledInput=0.0  OutMin=[]  OutMax=[]  OutDataType=fixdt(1, 16)  OutScaling=2^-10  DoSatur=off
  DocBlock : simulink/Model-Wide Utilities/DocBlock  DocumentType=Text
      content=|
      | For each wing section, things that need to be specified includes:
      | - Wing solid dimension (use wing modify script)
      | - Wing joint gain (pitchGain, pitchGain1, pitchGain2)
      | - PivotXfm & COMXfm
      | - i value
      | - inboard_yes?
  In_yes : Constant  Value=0
  Product : Product
  Switch : Switch  Criteria=u2 > Threshold  SaturateOnIntegerOverflow=off  InputSameDT=off
  WingSolid : sm_lib/Body Elements/Brick Solid  BrickDimensions=[0.25667, L_t, SectionWidth_Out]  BrickDimensionsUnits=m  ExportEntireGeometry=off  InertiaType=CalculateFromGeometry  BasedOnType=Mass  Density=1000  DensityUnits=kg/m^3  Mass=0.023048  MassUnits=kg  CenterOfMass=[0 0 0]  CenterOfMassUnits=m  MomentsOfInertia=[1 1 1]  MomentsOfInertiaUnits=kg*m^2  ProductsOfInertia=[0 0 0]  ProductsOfInertiaUnits=kg*m^2  GraphicType=FromGeometry  MarkerShape=Sphere  MarkerSize=10  GraphicVisPropType=SimpleVisualProperties  GraphicDiffuseColor=[0.65 0.4 0.8]  GraphicOpacity=1  GraphicSpecularColor=[0.5 0.5 0.5 1.0]  GraphicAmbientColor=[0.15 0.15 0.15 1.0]  GraphicEmissiveColor=[0.0 0.0 0.0 1.0]  GraphicShininess=75  DoExposeReferenceFrame=on  SerializedFrames=<Frames/>
  Wing_Joint : sm_lib/Joints/Revolute Joint  JointMode=Normal  CompositeWrenchDir=FollowerOnBase  CompositeWrenchFrame=BaseFrame  SenseConstraintForce=off  SenseConstraintTorque=off  SenseTotalForce=off  SenseTotalTorque=off  PositionTargetSpecify=off  PositionTargetPriority=High  PositionTargetValue=0  PositionTargetValueUnits=deg  VelocityTargetSpecify=off  VelocityTargetPriority=High  VelocityTargetValue=0  VelocityTargetValueUnits=deg/s  EquilibriumPosition=0  EquilibriumPositionUnits=deg  SpringStiffness=0  SpringStiffnessUnits=N*m/deg  DampingCoefficient=dampingOfJoints  DampingCoefficientUnits=N*m/(deg/s)  LowerLimitSpecify=off  LowerLimitBound=-90  LowerLimitBoundUnits=deg  LowerLimitStiffness=1e4  LowerLimitStiffnessUnits=N*m/deg  LowerLimitDamping=10  LowerLimitDampingUnits=N*m/(deg/s)  LowerLimitTransitionRegionWidth=0.1  LowerLimitTransitionRegionWidthUnits=deg  UpperLimitSpecify=off  UpperLimitBound=90  UpperLimitBoundUnits=deg  UpperLimitStiffness=1e4  UpperLimitStiffnessUnits=N*m/deg  UpperLimitDamping=10  UpperLimitDampingUnits=N*m/(deg/s)  UpperLimitTransitionRegionWidth=0.1  UpperLimitTransitionRegionWidthUnits=deg  TorqueActuationMode=ComputedTorque  MotionActuationMode=InputMotion  SensePosition=off  SenseVelocity=off  SenseAcceleration=off  SenseTorqueForce=off  SenseLowerLimitTorqueForce=off  SenseUpperLimitTorqueForce=off
  Xfm : sm_lib/Frames and Transforms/Rigid Transform  RotationMethod=None  FollAlignAxisA=+X  BaseAlignAxisA=+Y  FollAlignAxisB=+Y  BaseAlignAxisB=+Z  RotationStandardAxis=+Z  RotationAngle=0  RotationAngleUnits=deg  RotationArbitraryAxis=[0 0 1]  RotationSequenceAxes=FollowerAxes  RotationSequence=XYX  RotationSequenceAngles=[0 0 0]  RotationSequenceAnglesUnits=deg  RotationMatrix=[1 0 0;0 1 0;0 0 1]  Quaternion=[1 0 0 0]  TranslationMethod=Cartesian  TranslationCartesianOffset=[0.064167 0 0.27]  TranslationCartesianOffsetUnits=m  TranslationStandardAxis=+Z  TranslationStandardOffset=0  TranslationStandardOffsetUnits=m  TranslationROffset=0  TranslationROffsetUnits=m  TranslationThetaOffset=0  TranslationThetaOffsetUnits=deg  TranslationZOffset=0  TranslationZOffsetUnits=m
  i : Constant  Value=5
  pitchGain : Gain  Gain=0.5
  pitchGain1 : Gain  Gain=0.5
  pitchGain2 : Gain  Gain=0.5
  pitchPS : nesl_utility/Simulink-PS Converter  PhysicalDomain=network_engine_domain  SubClassName=ps_input  LeftPortType=input  RightPortType=output  PseudoPeriodic=off  Frequencies=[]  NoiseDistribution=none  NoiseParameters=[]  Unit=rad  AffineConversion=off  FilteringAndDerivatives=provide  SimscapeFilterOrder=1  InputFilterTimeConstant=0.001  UdotUserProvided=2
  pitch_lookup?(1=yes) : Constant  Value=pitch_lookup_input
  pitch_tip_in : FromWorkspace  VariableName=pitch_tip_in  SampleTime=del_t
  simulation sign convention differ : Constant  Value=-1
  WingRef_Frame : PMIOPort  Side=Left
  dL : Outport
  dT : Outport  Port=2
  wires:
  pitch_tip_in/1 -> Switch/3  "pitch"
  [pitch_m] -> Switch/1
  Switch/1 -> Product/1
  pitch_lookup?(1=yes)/1 -> Switch/2
  Product/1 -> pitchGain/1, Discrete Derivative/1
  simulation sign convention differ/1 -> Product/2
  In_yes/1 -> 1993dL&dT/2(inboard_yes?)
  i/1 -> 1993dL&dT/1(i)
  1993dL&dT/2(dT) -> dT/1
  Discrete Derivative/1 -> pitchGain1/1, Discrete Derivative1/1
  pitchGain/1 -> pitchPS/1
  1993dL&dT/1(dL) -> dL/1
  pitchGain2/1 -> pitchPS/3
  Discrete Derivative1/1 -> pitchGain2/1  "acc"
  pitchGain1/1 -> pitchPS/2
  connections:
  Xfm/LConn1 -- Wing_Joint/RConn1
  1993dL&dT/LConn1 -- Xfm/RConn1 -- WingSolid/RConn1
  pitchPS/RConn1 -- Wing_Joint/LConn2
  Wing_Joint/LConn1 -- WingRef_Frame/RConn1

== system LinkageC/Subsystem/Wing Tip/WingSeg_Out_6 ==
  1993dL&dT : Subsystem
      settings: PortSchema="{\"entries\":[{\"content\":{\"sides\":[{\"content\":{\"connectorIds\":[\"In1\",\"In2\"]},\"type\":\"ConnectorPlacement.EquallySpacedRectSide\",\"uuid\":\"e65777f2-64e1-48f2-8a97-1c4430d49e8c\"},{\"content\":{\"connectorIds\":[\"Out1\",\"Out2\"],\"side\":\"RIGHT\"},\"type\":\"ConnectorPlacement.EquallySpacedRectSide\",\"uuid\":\"b36152b1-49d2-4fe8-8958-784e9c481724\"},{\"content\":{\"connectorIds\":[\"LConn1\"],\"side\":\"TOP\"},\"type\":\"ConnectorPlacement.EquallySpacedRectSide\",\"uuid\":\"e55ca923-aa34-4679-961a-c06571c550d8\"}]},\"type\":\"ConnectorPlacement.EquallySpacedConnector\",\"uuid\":\"74bedadb-397c-4a7f-b538-7cebaf15bb03\"}],\"packageUris\":[\"http://schema.mathworks.com/mf0/Connector/R2020b\"],\"version\":\"1.0\"}"
  Discrete Derivative : simulink/Discrete/Discrete Derivative  gainval=1.0  ICPrevScaledInput=0.0  OutMin=[]  OutMax=[]  OutDataType=fixdt(1, 16)  OutScaling=2^-10  DoSatur=off
  Discrete Derivative1 : simulink/Discrete/Discrete Derivative  gainval=1.0  ICPrevScaledInput=0.0  OutMin=[]  OutMax=[]  OutDataType=fixdt(1, 16)  OutScaling=2^-10  DoSatur=off
  DocBlock : simulink/Model-Wide Utilities/DocBlock  DocumentType=Text
      content=|
      | For each wing section, things that need to be specified includes:
      | - Wing solid dimension (use wing modify script)
      | - Wing joint gain (pitchGain, pitchGain1, pitchGain2)
      | - PivotXfm & COMXfm
      | - i value
      | - inboard_yes?
  In_yes : Constant  Value=0
  Product : Product
  Switch : Switch  Criteria=u2 > Threshold  SaturateOnIntegerOverflow=off  InputSameDT=off
  WingSolid : sm_lib/Body Elements/Brick Solid  BrickDimensions=[0.23333, L_t, SectionWidth_Out]  BrickDimensionsUnits=m  ExportEntireGeometry=off  InertiaType=CalculateFromGeometry  BasedOnType=Mass  Density=1000  DensityUnits=kg/m^3  Mass=0.020952  MassUnits=kg  CenterOfMass=[0 0 0]  CenterOfMassUnits=m  MomentsOfInertia=[1 1 1]  MomentsOfInertiaUnits=kg*m^2  ProductsOfInertia=[0 0 0]  ProductsOfInertiaUnits=kg*m^2  GraphicType=FromGeometry  MarkerShape=Sphere  MarkerSize=10  GraphicVisPropType=SimpleVisualProperties  GraphicDiffuseColor=[0.72 0.4 0.8]  GraphicOpacity=1  GraphicSpecularColor=[0.5 0.5 0.5 1.0]  GraphicAmbientColor=[0.15 0.15 0.15 1.0]  GraphicEmissiveColor=[0.0 0.0 0.0 1.0]  GraphicShininess=75  DoExposeReferenceFrame=on  SerializedFrames=<Frames/>
  Wing_Joint : sm_lib/Joints/Revolute Joint  JointMode=Normal  CompositeWrenchDir=FollowerOnBase  CompositeWrenchFrame=BaseFrame  SenseConstraintForce=off  SenseConstraintTorque=off  SenseTotalForce=off  SenseTotalTorque=off  PositionTargetSpecify=off  PositionTargetPriority=High  PositionTargetValue=0  PositionTargetValueUnits=deg  VelocityTargetSpecify=off  VelocityTargetPriority=High  VelocityTargetValue=0  VelocityTargetValueUnits=deg/s  EquilibriumPosition=0  EquilibriumPositionUnits=deg  SpringStiffness=0  SpringStiffnessUnits=N*m/deg  DampingCoefficient=dampingOfJoints  DampingCoefficientUnits=N*m/(deg/s)  LowerLimitSpecify=off  LowerLimitBound=-90  LowerLimitBoundUnits=deg  LowerLimitStiffness=1e4  LowerLimitStiffnessUnits=N*m/deg  LowerLimitDamping=10  LowerLimitDampingUnits=N*m/(deg/s)  LowerLimitTransitionRegionWidth=0.1  LowerLimitTransitionRegionWidthUnits=deg  UpperLimitSpecify=off  UpperLimitBound=90  UpperLimitBoundUnits=deg  UpperLimitStiffness=1e4  UpperLimitStiffnessUnits=N*m/deg  UpperLimitDamping=10  UpperLimitDampingUnits=N*m/(deg/s)  UpperLimitTransitionRegionWidth=0.1  UpperLimitTransitionRegionWidthUnits=deg  TorqueActuationMode=ComputedTorque  MotionActuationMode=InputMotion  SensePosition=off  SenseVelocity=off  SenseAcceleration=off  SenseTorqueForce=off  SenseLowerLimitTorqueForce=off  SenseUpperLimitTorqueForce=off
  Xfm : sm_lib/Frames and Transforms/Rigid Transform  RotationMethod=None  FollAlignAxisA=+X  BaseAlignAxisA=+Y  FollAlignAxisB=+Y  BaseAlignAxisB=+Z  RotationStandardAxis=+Z  RotationAngle=0  RotationAngleUnits=deg  RotationArbitraryAxis=[0 0 1]  RotationSequenceAxes=FollowerAxes  RotationSequence=XYX  RotationSequenceAngles=[0 0 0]  RotationSequenceAnglesUnits=deg  RotationMatrix=[1 0 0;0 1 0;0 0 1]  Quaternion=[1 0 0 0]  TranslationMethod=Cartesian  TranslationCartesianOffset=[0.058333 0 0.33]  TranslationCartesianOffsetUnits=m  TranslationStandardAxis=+Z  TranslationStandardOffset=0  TranslationStandardOffsetUnits=m  TranslationROffset=0  TranslationROffsetUnits=m  TranslationThetaOffset=0  TranslationThetaOffsetUnits=deg  TranslationZOffset=0  TranslationZOffsetUnits=m
  i : Constant  Value=6
  pitchGain : Gain  Gain=0.6
  pitchGain1 : Gain  Gain=0.6
  pitchGain2 : Gain  Gain=0.6
  pitchPS : nesl_utility/Simulink-PS Converter  PhysicalDomain=network_engine_domain  SubClassName=ps_input  LeftPortType=input  RightPortType=output  PseudoPeriodic=off  Frequencies=[]  NoiseDistribution=none  NoiseParameters=[]  Unit=rad  AffineConversion=off  FilteringAndDerivatives=provide  SimscapeFilterOrder=1  InputFilterTimeConstant=0.001  UdotUserProvided=2
  pitch_lookup?(1=yes) : Constant  Value=pitch_lookup_input
  pitch_tip_in : FromWorkspace  VariableName=pitch_tip_in  SampleTime=del_t
  simulation sign convention differ : Constant  Value=-1
  WingRef_Frame : PMIOPort  Side=Left
  dL : Outport
  dT : Outport  Port=2
  wires:
  pitch_tip_in/1 -> Switch/3  "pitch"
  [pitch_m] -> Switch/1
  Switch/1 -> Product/1
  pitch_lookup?(1=yes)/1 -> Switch/2
  Product/1 -> pitchGain/1, Discrete Derivative/1
  simulation sign convention differ/1 -> Product/2
  In_yes/1 -> 1993dL&dT/2(inboard_yes?)
  i/1 -> 1993dL&dT/1(i)
  1993dL&dT/2(dT) -> dT/1
  Discrete Derivative/1 -> pitchGain1/1, Discrete Derivative1/1
  pitchGain/1 -> pitchPS/1
  1993dL&dT/1(dL) -> dL/1
  pitchGain2/1 -> pitchPS/3
  Discrete Derivative1/1 -> pitchGain2/1  "acc"
  pitchGain1/1 -> pitchPS/2
  connections:
  Xfm/LConn1 -- Wing_Joint/RConn1
  1993dL&dT/LConn1 -- Xfm/RConn1 -- WingSolid/RConn1
  pitchPS/RConn1 -- Wing_Joint/LConn2
  Wing_Joint/LConn1 -- WingRef_Frame/RConn1
